simulink model "mission"  (R2019a)
settings: Solver=ode8  StartTime=0.0  StopTime=10000  FixedStep=.1  MaxStep=30  MinStep=1  RelTol=1e-7
PreLoadFcn:
  | load('D:\OneDrive\IonSat X18\SCAO\SIMULINK\Data\SatConstants.mat')
model workspace (MAT data in the model file):
  repartition_matrix = Simulink.Parameter
  repartition_matrix.DataType = 'auto'
  repartition_matrix.Dimensions = [0 0]
  wheel_number = Simulink.Parameter
  wheel_number.Value = 3
  wheel_number.DataType = 'auto'
  wheel_number.Dimensions = [1 1]
undefined symbols (not defined in the file or in its folder): deg, IAU, km, m, mu_Earth, rad, s, sat, X, Y, Z
libraries: sm_lib x19, nesl_utility x16, aerolibutil x15, aerolibconvert2 x12, dspmathops x8, vrlib x5, sharedtransform x5, sharedutil x4, aerolibtransform2 x2, aerolibgravity2 x2, simulink x1, aerolibcelestial x1
(part 1 of 3)
settings Model: SnapshotBufferSize=100  OrderedModelArguments=off  Creator=robin  LastModifiedBy=brice
settings SolverCC: InitialStep=1
settings DataIOCC: SaveFormat=StructureWithTime  SaveOutput=off  SignalLogging=off  DSMLogging=off  SaveTime=off
settings OptimizationCC: DefaultParameterBehavior=Inlined  UseDivisionForNetSlopeComputation=on  GainParamInheritBuiltInType=on  UseFloatMulNetSlope=on  InlineInvariantSignals=on  PassReuseOutputArgsAs=Individual arguments  ZeroExternalMemoryAtStartup=off  ZeroInternalMemoryAtStartup=off  NoFixptDivByZeroProtection=on  EfficientFloat2IntCast=on  LifeSpan=1  OptimizeBlockOrder=speed  DifferentSizesBufferReuse=on
settings DebuggingCC: ParameterTunabilityLossMsg=error
settings HardwareCC: ProdBitPerInt=16  ProdBitPerPointer=8  ProdBitPerSizeT=24  ProdBitPerPtrDiffT=24  ProdLargestAtomicFloat=None  ProdWordSize=8  ProdLongLongMode=on  ProdHWDeviceType=Microchip->PIC18
settings SFSimCC: MATLABDynamicMemAlloc=off
settings RTWCC: SystemTargetFile=ert.tlc  TemplateMakefile=ert_default_tmf  GenerateReport=on  IncludeHyperlinkInReport=on  LaunchReport=on  GenerateTraceInfo=on  GenerateTraceReport=on  GenerateTraceReportSl=on  GenerateTraceReportSf=on  GenerateTraceReportEml=on  GenerateCodeMetricsReport=on
settings CodeAppCC: ForceParamTrailComments=on  IgnoreCustomStorageClasses=off  OperatorAnnotations=on  SimulinkDataObjDesc=on  SFDataObjDesc=on  CustomSymbolStrGlobalVar=rt$N$M  CustomSymbolStrType=$N$M  CustomSymbolStrFcn=$N$M$F  CustomSymbolStrMacro=$N$M  InsertBlockDesc=on
settings ERTTargetCC: TargetLangStandard=C99 (ISO)  GenerateSampleERTMain=on  IncludeMdlTerminateFcn=off  CombineSignalStateStructs=on  SupportAbsoluteTime=off  SupportComplex=off  SupportContinuousTime=on  SupportNonInlinedSFcns=on  InlinedParameterPlacement=NonHierarchical  ERTCustomFileTemplate=example_file_process.tlc  ERTFilePackagingFormat=CompactWithDataFile

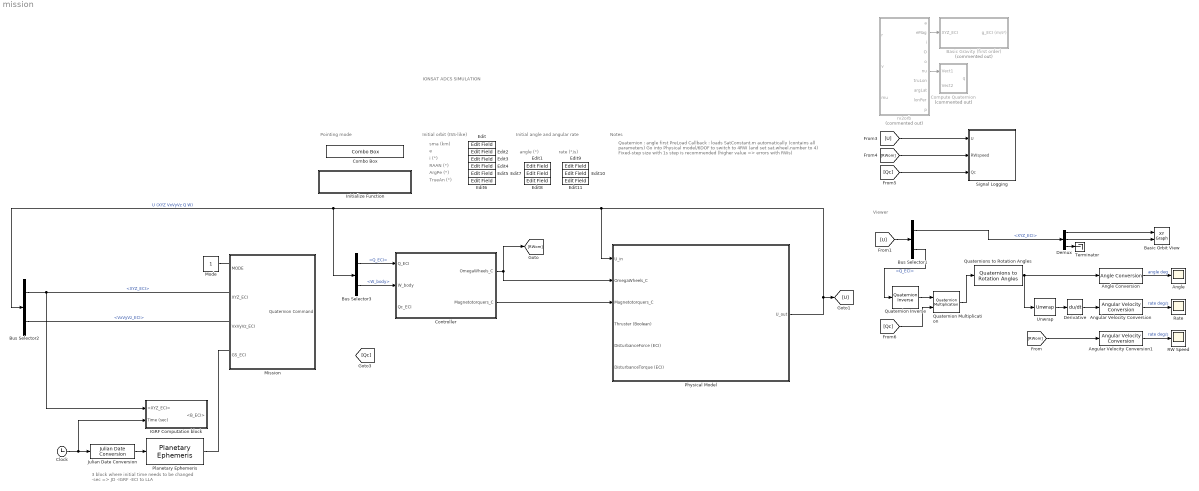
== system mission ==
  note: 3 block where initial time needs to be changed
      | -sec => JD
      | -IGRF
      | -ECI to LLA
  note: IONSAT ADCS SIMULATION
  note: Viewer
  note: Pointing mode
  note: Initial orbit (ISS-like)
  note: sma (km)
  note: e
  note: i (°)
  note: RAAN (°)
  note: ArgPe (°)
  note: TrueAn (°)
  note: Initial angle and angular rate
  note: angle (°)
  note: rate (°/s)
  note: Notes
  note: Quaternion : angle first
      | PreLoad Callback : loads SatConstant.m automatically (contains all parameters)
      | Go into Physical model/6DOF to switch to 4RW (and set sat.wheel.number to 4)
      | Fixed-step size with 1s step is recommended (higher value => errors with RWs)
  Angle : Scope
  Angle Conversion : aerolibconvert2/Angle Conversion  IU=rad  OU=deg
  Angular Velocity Conversion : aerolibconvert2/Angular Velocity Conversion  IU=rad/s  OU=deg/s
      settings: SourceProductName=Aerospace Blockset
  Angular Velocity Conversion1 : aerolibconvert2/Angular Velocity Conversion  IU=rad/s  OU=deg/s
      settings: SourceProductName=Aerospace Blockset
  Basic Gravity (first order) : Subsystem  Commented=on
  Basic Orbit View : simulink/Sinks/XY Graph  xmin=-10000000  xmax=10000000  ymin=-10000000  ymax=10000000  st=-1
  Bus Selector1 : BusSelector  OutputSignals=XYZ_ECI,Q_ECI
  Bus Selector2 : BusSelector  OutputSignals=XYZ_ECI,VxVyVz_ECI
  Bus Selector3 : BusSelector  OutputSignals=Q_ECI,W_body
  Clock : Clock
  Combo Box : ComboBox  LabelPosition=Hide  SelectedLabel=Nadir
      settings: Values={{'Nadir', 'Retrograde', 'Drag', 'Sun', 'Sun Aero'}, [1 5 4 3 2]}
  Compute Quaternion : Subsystem  Commented=on
  Controller : Subsystem  TreatAsAtomicUnit=on  SystemSampleTime=1
  Demux : Demux  Outputs=3
  Derivative : Derivative
  Edit{,1..11} (12 alike) : EditField  LabelPosition=Hide  ShowInitialText=on  Alignment=Center
  IGRF Computation block : Subsystem
  Initialize Function : Subsystem  TreatAsAtomicUnit=on
  Julian Date Conversion : aerolibconvert2/Julian Date Conversion  year=2020  month=January  day=1  hour=0  min=0  sec=0  modflag=off  deltaT=Sec  errorflag=Error
      settings: SourceProductName=Aerospace Blockset  SourceProductBaseCode=AE
  Mission : Subsystem  TreatAsAtomicUnit=on  SystemSampleTime=1
  Mode : Constant  OutDataTypeStr=int8
  Physical Model : Subsystem
  Planetary Ephemeris : aerolibcelestial/Planetary Ephemeris  kmflag=km,km/s  epochflag=Julian date  de=DE405  nCenter=Earth  nTarget=Sun  errorflag=Error  velflag=off
      settings: AttributesFormatString=Ephemeris Data Unavailable  SourceProductName=Aerospace Blockset  SourceProductBaseCode=AE
  Quaternion Inverse : aerolibutil/Quaternion Inverse
      settings: SourceProductName=Aerospace Blockset
  Quaternion Multiplication : aerolibutil/Quaternion Multiplication
  Quaternions to Rotation Angles : sharedtransform/Quaternions to Rotation Angles  rotationOrder=ZYX  aMode=aMode
      settings: SourceProductBaseCode=AE
  RW Speed : Scope
  Rate : Scope
  Signal Logging : Subsystem
  Terminator : Terminator
  Unwrap : dspsigops/Unwrap  tol=pi  running=off
  rv2orb : MATLAB Function  Commented=on  TreatAsAtomicUnit=on
  wires:
  ? -> [Qc], Controller/3(Qc_ECI)  "Quaternion Command"
  Mode/1 -> ?
  Bus Selector2/2 -> ?  "<VxVyVz_ECI>"
  Physical Model/1(U_out) -> Bus Selector3/1, Bus Selector2/1, Physical Model/1(U_in), [U]  "U (XYZ VxVyVz Q W)"
  Controller/2(Magnetotorquers_C) -> Physical Model/3(Magnetotorquers_C)
  Controller/1(OmegaWheels_C) -> [RWom], Physical Model/2(OmegaWheels_C)
  Angle Conversion/1 -> Angle/1  "angle deg"
  Demux/3 -> Terminator/1
  Demux/2 -> Basic Orbit View/2
  Angular Velocity Conversion/1 -> Rate/1  "rate deg/s"
  Bus Selector1/1 -> Demux/1  "<XYZ_ECI>"
  Quaternion Multiplication/1 -> Quaternions to Rotation Angles/1
  Demux/1 -> Basic Orbit View/1
  Derivative/1 -> Angular Velocity Conversion/1
  Quaternions to Rotation Angles/1 -> Unwrap/1, Angle Conversion/1
  Unwrap/1 -> Derivative/1
  Angular Velocity Conversion1/1 -> RW Speed/1  "rate deg/s"
  [RWom] -> Angular Velocity Conversion1/1
  [U] -> Bus Selector1/1
  rv2orb/2(eMag) -> Basic Gravity (first order)/1(XYZ_ECI)
  Bus Selector2/1 -> IGRF Computation block/1(<XYZ_ECI>)  "<XYZ_ECI>"
  rv2orb/6(nu) -> Compute Quaternion/1(Vect1)
  Bus Selector3/1 -> Controller/1(Q_ECI)  "<Q_ECI>"
  Bus Selector3/2 -> Controller/2(W_body)  "<W_body>"
  Julian Date Conversion/1 -> Planetary Ephemeris/1
  Clock/1 -> Julian Date Conversion/1, IGRF Computation block/2(Time (sec))
  Planetary Ephemeris/1 -> ?
  [U] -> Signal Logging/1(U)
  [RWom] -> Signal Logging/2(RWspeed)
  [Qc] -> Signal Logging/3(Qc)
  [Qc] -> Quaternion Multiplication/2
  Quaternion Inverse/1 -> Quaternion Multiplication/1
  Bus Selector1/2 -> Quaternion Inverse/1  "<Q_ECI>"

== system mission/Basic Gravity (first order) ==
  XYZ_ECI : Inport
  Constant : Constant  Value=-mu_Earth
  Constant3 : Constant  Value=3/2
  Divide : Product  Inputs=*/
  Norm : Subsystem
  Product : Product
  Square3 : Math  Operator=pow  SaturateOnIntegerOverflow=on
  g_ECI (m/s²) : Outport  VectorParamsAs1DForOutWhenUnconnected=on
  wires:
  Constant/1 -> Divide/1
  Divide/1 -> Product/2
  Product/1 -> g_ECI (m/s²)/1
  XYZ_ECI/1 -> Norm/1(u), Product/1
  Square3/1 -> Divide/2  "r**3"
  Constant3/1 -> Square3/2
  Norm/1(r**2) -> Square3/1

== system mission/Compute Quaternion ==
  Vect1 : Inport
  Vect2 : Inport  Port=2
  Constant : Constant
  Cross Product : vrlib/Utilities/Cross Product
      settings: SourceProductName=Simulink
  Dot Product : DotProduct  InputSameDT=on  OutDataTypeStr=Inherit: Inherit via internal rule
  Mux : Mux  Inputs=2
  Normalization : dspmathops/Normalization  NormType=2-norm  Bias=1e-10  NormOver=Each column  Dimension=1  roundingMode=Floor  overflowMode=off  accumDataTypeStr=Inherit: Same as product output  accumLastDataTypeStr=Inherit: Same as product output  outputDataTypeStr=Inherit: Same as product output  outputMin=[]  outputMax=[]  outputLastDataTypeStr=Inherit: Same as product output
      settings: SourceProductName=DSP System Toolbox
  Normalization1 : dspmathops/Normalization  NormType=2-norm  Bias=1e-10  NormOver=Each column  Dimension=1  roundingMode=Floor  overflowMode=off  accumDataTypeStr=Inherit: Same as product output  accumLastDataTypeStr=Inherit: Same as product output  outputDataTypeStr=Inherit: Same as product output  outputMin=[]  outputMax=[]  outputLastDataTypeStr=Inherit: Same as product output
      settings: SourceProductName=DSP System Toolbox
  Quaternion Normalize : sharedutil/Quaternion Normalize  aMode=aMode
      settings: SourceProductName=Aerospace Blockset  SourceProductBaseCode=AE
  Sum : Sum  Inputs=|++
  q : Outport  PortDimensions=4
  wires:
  Vect1/1 -> Normalization/1
  Normalization/1 -> Cross Product/1, Dot Product/1
  Vect2/1 -> Normalization1/1
  Normalization1/1 -> Dot Product/2, Cross Product/2
  Cross Product/1 -> Mux/2
  Dot Product/1 -> Sum/1
  Sum/1 -> Mux/1
  Constant/1 -> Sum/2
  Mux/1 -> Quaternion Normalize/1
  Quaternion Normalize/1 -> q/1

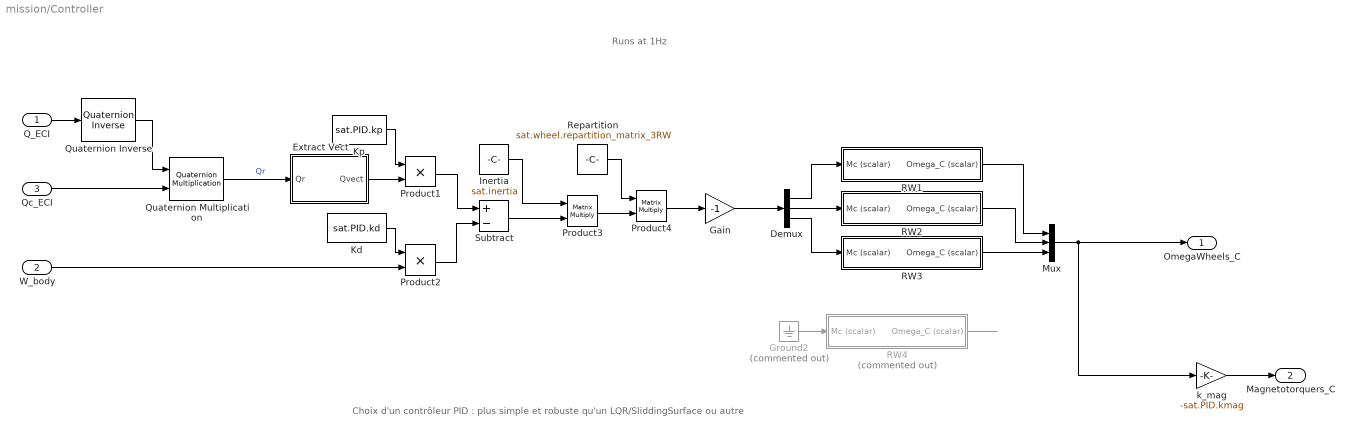
== system mission/Controller ==
  note: Choix d'un contrôleur PID : plus simple et robuste qu'un LQR/SliddingSurface ou autre
  note: Runs at 1Hz
  Q_ECI : Inport
  W_body : Inport  Port=2
  Qc_ECI : Inport  Port=3
  Demux : Demux  Outputs=3
  Extract Vect : Subsystem
  Gain : Gain  Gain=-1
  Ground2 : Ground  Commented=on
  Inertia : Constant  Value=sat.inertia
  Kd : Constant  Value=sat.PID.kd
  Kp : Constant  Value=sat.PID.kp
  Mux : Mux  Inputs=3
  Product1 : Product
  Product2 : Product
  Product3 : Product  Multiplication=Matrix(*)
  Product4 : Product  Multiplication=Matrix(*)
  Quaternion Inverse : aerolibutil/Quaternion Inverse
      settings: SourceProductName=Aerospace Blockset
  Quaternion Multiplication : aerolibutil/Quaternion Multiplication
  RW1 : Subsystem
  RW2 : Subsystem
  RW3 : Subsystem
  RW4 : Subsystem  Commented=on
  Repartition : Constant  Value=sat.wheel.repartition_matrix_3RW
  Subtract : Sum  Inputs=+-
  k_mag : Gain  Gain=-sat.PID.kmag
  OmegaWheels_C : Outport
  Magnetotorquers_C : Outport  Port=2
  wires:
  RW1/1(Omega_C (scalar)) -> Mux/1
  RW2/1(Omega_C (scalar)) -> Mux/2
  RW3/1(Omega_C (scalar)) -> Mux/3
  RW4/1(Omega_C (scalar)) -> ?
  Demux/3 -> RW3/1(Mc (scalar))
  Ground2/1 -> RW4/1(Mc (scalar))
  Qc_ECI/1 -> Quaternion Multiplication/2
  Quaternion Multiplication/1 -> Extract Vect/1(Qr)  "Qr"
  Kp/1 -> Product1/1
  Extract Vect/1(Qvect) -> Product1/2
  W_body/1 -> Product2/2
  Kd/1 -> Product2/1
  Product2/1 -> Subtract/2
  Product1/1 -> Subtract/1
  Subtract/1 -> Product3/2
  Inertia/1 -> Product3/1
  Product3/1 -> Product4/2
  Repartition/1 -> Product4/1
  Demux/2 -> RW2/1(Mc (scalar))
  Demux/1 -> RW1/1(Mc (scalar))
  Product4/1 -> Gain/1
  Q_ECI/1 -> Quaternion Inverse/1
  Quaternion Inverse/1 -> Quaternion Multiplication/1
  Gain/1 -> Demux/1
  k_mag/1 -> Magnetotorquers_C/1
  Mux/1 -> k_mag/1, OmegaWheels_C/1

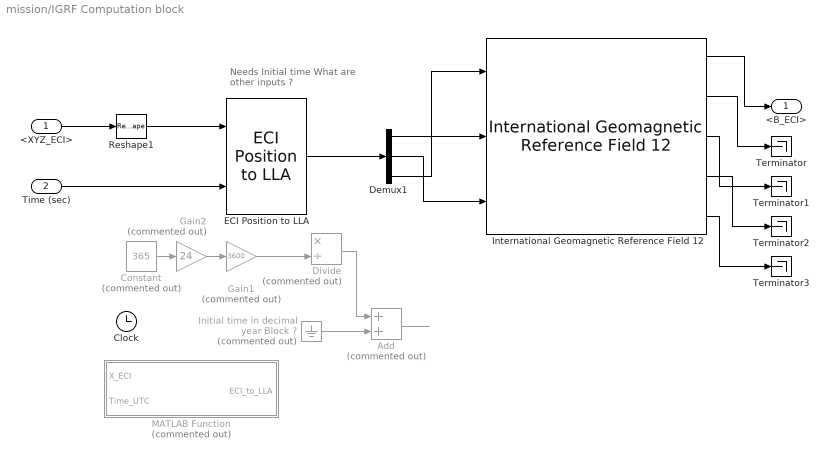
== system mission/IGRF Computation block ==
  note: Needs Initial time
      | What are other inputs ?
  <XYZ_ECI> : Inport
  Time (sec) : Inport  Port=2
  Add : Sum  Commented=on
  Clock : Clock
  Constant : Constant  Commented=on  Value=365
  Demux1 : Demux  Outputs=3
  Divide : Product  Commented=on  Inputs=*/
  ECI Position to LLA : aerolibtransform2/ECI Position to LLA  red=IAU-2000/2006  year=2020  month=January  day=1  hour=0  min=0  sec=0  deltaT=Sec  errorflag=Error  extraparamflag=off  eunits=Metric (MKS)  earthmodel=WGS84  flat=1/298.257223563  eqradius=6378137
      settings: AttributesFormatString=%<red>  SourceProductName=Aerospace Blockset  SourceProductBaseCode=AE
  Gain1 : Gain  Commented=on  Gain=3600
  Gain2 : Gain  Commented=on  Gain=24
  Initial time in decimal year Block ? : Ground  Commented=on
  International Geomagnetic Reference Field 12 : aerolibgravity2/International Geomagnetic Reference Field 12  units=Metric (MKS)  time_in=off  month=January  day=1  year=2020  action=None  sv_out=off
      settings: SourceProductName=Aerospace Blockset  SourceProductBaseCode=AE
  MATLAB Function : MATLAB Function  Commented=on  TreatAsAtomicUnit=on
  Reshape1 : Reshape  OutputDimensionality=Column vector (2-D)
  Terminator{,1..3} (4 alike) : Terminator
  <B_ECI> : Outport
  wires:
  International Geomagnetic Reference Field 12/1 -> <B_ECI>/1
  Demux1/2 -> International Geomagnetic Reference Field 12/3
  Time (sec)/1 -> ECI Position to LLA/2
  ECI Position to LLA/1 -> Demux1/1
  <XYZ_ECI>/1 -> Reshape1/1
  Gain2/1 -> Gain1/1
  Constant/1 -> Gain2/1
  Gain1/1 -> Divide/2
  Add/1 -> ?
  Divide/1 -> Add/1
  Initial time in decimal year Block ?/1 -> Add/2
  Reshape1/1 -> ECI Position to LLA/1
  International Geomagnetic Reference Field 12/3 -> Terminator1/1
  International Geomagnetic Reference Field 12/2 -> Terminator/1
  International Geomagnetic Reference Field 12/4 -> Terminator2/1
  International Geomagnetic Reference Field 12/5 -> Terminator3/1
  Demux1/1 -> International Geomagnetic Reference Field 12/2
  Demux1/3 -> International Geomagnetic Reference Field 12/1

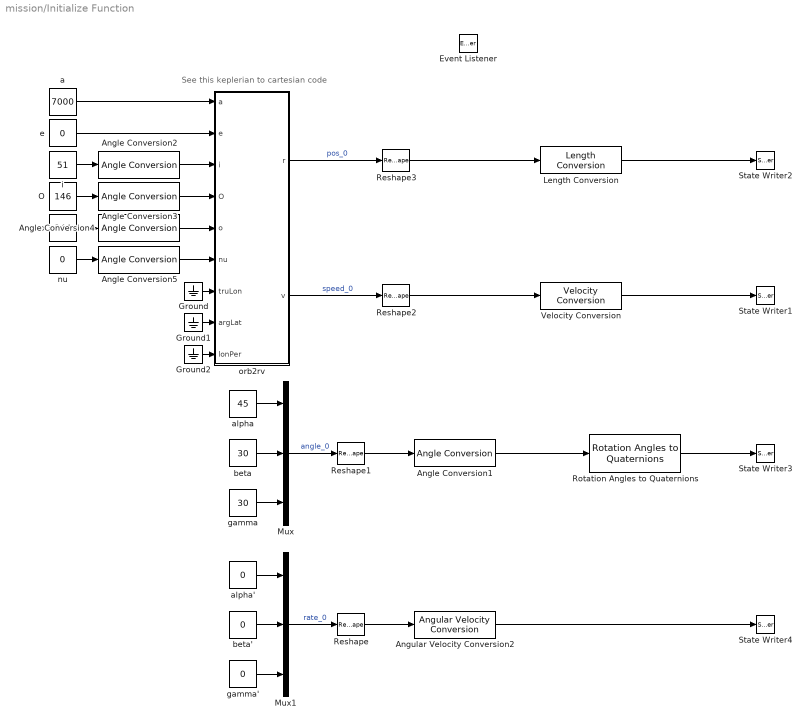
== system mission/Initialize Function ==
  note: See this keplerian to cartesian code
  Angle Conversion{1..5} (5 alike) : aerolibconvert2/Angle Conversion  IU=deg  OU=rad
  Angular Velocity Conversion2 : aerolibconvert2/Angular Velocity Conversion  IU=deg/s  OU=rad/s
      settings: SourceProductName=Aerospace Blockset
  Event Listener : EventListener  DisableCoverage=on  EventName=reset
  Ground : Ground
  Ground1 : Ground
  Ground2 : Ground
  Length Conversion : aerolibconvert2/Length Conversion  IU=km  OU=m
  Mux : Mux  Inputs=3
  Mux1 : Mux  Inputs=3
  O : Constant  Value=146
  Reshape{,1..3} (4 alike) : Reshape  OutputDimensionality=Column vector (2-D)
  Rotation Angles to Quaternions : sharedtransform/Rotation Angles to Quaternions  rotationOrder=ZYX  aMode=aMode
      settings: SourceProductName=Aerospace Blockset  SourceProductBaseCode=AE
  State Writer1 : StateWriter  StateOwnerBlock=../../Physical Model/6DOF in ECI frame/Integrator_speed
  State Writer2 : StateWriter  StateOwnerBlock=../../Physical Model/6DOF in ECI frame/Integrator_pos
  State Writer3 : StateWriter  StateOwnerBlock=../../Physical Model/6DOF in ECI frame/Compute Q_ECI/Integrator_quat
  State Writer4 : StateWriter  StateOwnerBlock=../../Physical Model/6DOF in ECI frame/Integrator_rate
  Velocity Conversion : aerolibconvert2/Velocity Conversion  IU=km/s  OU=m/s
  a : Constant  Value=7000
  alpha : Constant  Value=45
  alpha' : Constant  Value=0
  beta : Constant  Value=30
  beta' : Constant  Value=0
  e : Constant  Value=0
  gamma : Constant  Value=30
  gamma' : Constant  Value=0
  i : Constant  Value=51
  nu : Constant  Value=0
  o : Constant  Value=344
  orb2rv : MATLAB Function  TreatAsAtomicUnit=on
  wires:
  Angular Velocity Conversion2/1 -> State Writer4/1
  Angle Conversion1/1 -> Rotation Angles to Quaternions/1
  orb2rv/1(r) -> Reshape3/1  "pos_0"
  Mux1/1 -> Reshape/1  "rate_0"
  Mux/1 -> Reshape1/1  "angle_0"
  orb2rv/2(v) -> Reshape2/1  "speed_0"
  Rotation Angles to Quaternions/1 -> State Writer3/1
  Reshape/1 -> Angular Velocity Conversion2/1
  Reshape1/1 -> Angle Conversion1/1
  Reshape2/1 -> Velocity Conversion/1
  Reshape3/1 -> Length Conversion/1
  a/1 -> orb2rv/1(a)
  e/1 -> orb2rv/2(e)
  i/1 -> Angle Conversion2/1
  O/1 -> Angle Conversion3/1
  o/1 -> Angle Conversion4/1
  nu/1 -> Angle Conversion5/1
  Angle Conversion2/1 -> orb2rv/3(i)
  Angle Conversion3/1 -> orb2rv/4(O)
  Angle Conversion4/1 -> orb2rv/5(o)
  Angle Conversion5/1 -> orb2rv/6(nu)
  Ground/1 -> orb2rv/7(truLon)
  Ground1/1 -> orb2rv/8(argLat)
  Ground2/1 -> orb2rv/9(lonPer)
  Length Conversion/1 -> State Writer2/1
  Velocity Conversion/1 -> State Writer1/1
  alpha/1 -> Mux/1
  beta/1 -> Mux/2
  gamma/1 -> Mux/3
  alpha'/1 -> Mux1/1
  gamma'/1 -> Mux1/3
  beta'/1 -> Mux1/2

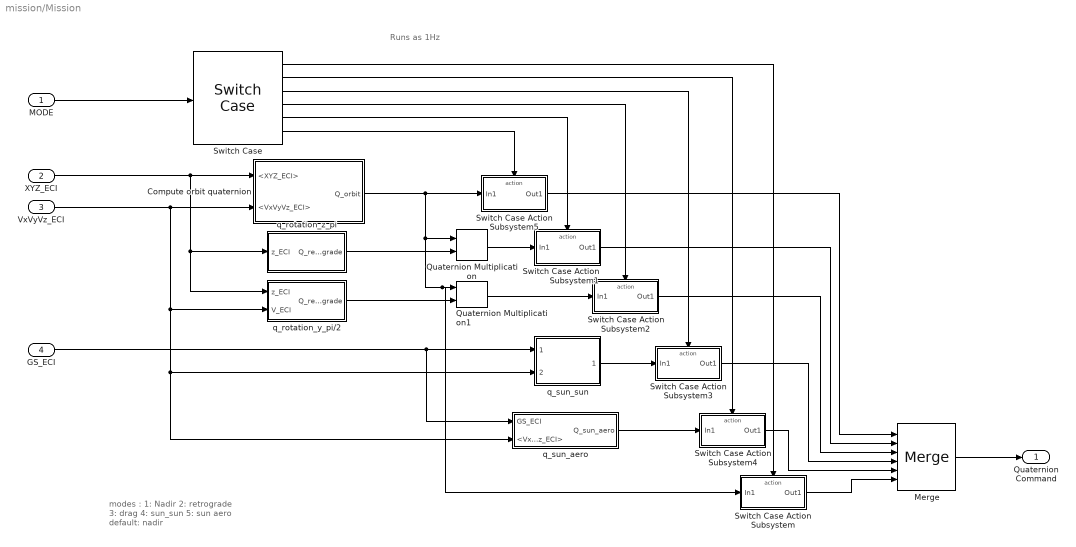
== system mission/Mission ==
  note: modes :
      | 1: Nadir
      | 2: retrograde
      | 3: drag
      | 4: sun_sun
      | 5: sun aero
      | default: nadir
  note: Runs as 1Hz
  MODE : Inport  OutMin=1  OutMax=100  OutDataTypeStr=int8
  XYZ_ECI : Inport  Port=2
  VxVyVz_ECI : Inport  Port=3
  GS_ECI : Inport  Port=4
  Compute orbit quaternion : Subsystem
  Merge : Merge  Inputs=6
  Quaternion Multiplication : aerolibutil/Quaternion Multiplication
  Quaternion Multiplication1 : aerolibutil/Quaternion Multiplication
  Switch Case : SwitchCase  CaseConditions={1, 2, 3, 4, 5}
  Switch Case Action Subsystem : Subsystem  TreatAsAtomicUnit=on
  Switch Case Action Subsystem1 : Subsystem  TreatAsAtomicUnit=on
  Switch Case Action Subsystem2 : Subsystem  TreatAsAtomicUnit=on
  Switch Case Action Subsystem3 : Subsystem  TreatAsAtomicUnit=on
  Switch Case Action Subsystem4 : Subsystem  TreatAsAtomicUnit=on
  Switch Case Action Subsystem5 : Subsystem  TreatAsAtomicUnit=on
  q_rotation_y_pi/2 : Subsystem
  q_rotation_z_pi : Subsystem
  q_sun_aero : Subsystem
  q_sun_sun : Subsystem
  Quaternion Command : Outport
  wires:
  q_rotation_y_pi/2/1(Q_retrograde) -> Quaternion Multiplication1/2
  Switch Case/6 -> Switch Case Action Subsystem5/Action
  Switch Case/3 -> Switch Case Action Subsystem3/Action
  Switch Case/1 -> Switch Case Action Subsystem/Action
  MODE/1 -> Switch Case/1
  Switch Case Action Subsystem2/1(Out1) -> Merge/3
  Switch Case Action Subsystem4/1(Out1) -> Merge/5
  Quaternion Multiplication1/1 -> Switch Case Action Subsystem2/1(In1)
  GS_ECI/1 -> q_sun_aero/1(GS_ECI), q_sun_sun/1(<VxVyVz_ECI>)
  Switch Case Action Subsystem3/1(Out1) -> Merge/4
  XYZ_ECI/1 -> q_rotation_y_pi/2/1(z_ECI), q_rotation_z_pi/1(z_ECI), Compute orbit quaternion/1(<XYZ_ECI>)
  Switch Case/4 -> Switch Case Action Subsystem2/Action
  Compute orbit quaternion/1(Q_orbit) -> Switch Case Action Subsystem/1(In1), Quaternion Multiplication1/1, Quaternion Multiplication/1, Switch Case Action Subsystem5/1(In1)
  Switch Case Action Subsystem/1(Out1) -> Merge/6
  Quaternion Multiplication/1 -> Switch Case Action Subsystem1/1(In1)
  q_rotation_z_pi/1(Q_retrograde) -> Quaternion Multiplication/2
  Switch Case/5 -> Switch Case Action Subsystem1/Action
  Switch Case Action Subsystem1/1(Out1) -> Merge/2
  q_sun_aero/1(Q_sun_aero) -> Switch Case Action Subsystem4/1(In1)
  Merge/1 -> Quaternion Command/1
  Switch Case/2 -> Switch Case Action Subsystem4/Action
  Switch Case Action Subsystem5/1(Out1) -> Merge/1
  q_sun_sun/1(Q_sun_sun) -> Switch Case Action Subsystem3/1(In1)
  VxVyVz_ECI/1 -> q_sun_aero/2(<VxVyVz_ECI>), q_sun_sun/2(GS_ECI), q_rotation_y_pi/2/2(V_ECI), Compute orbit quaternion/2(<VxVyVz_ECI>)

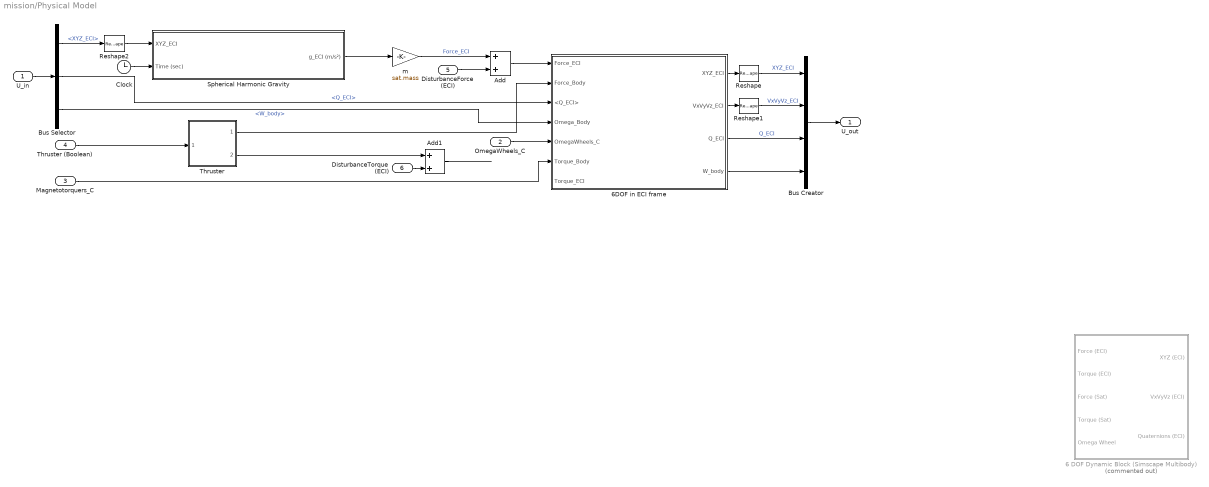
== system mission/Physical Model ==
  U_in : Inport
  OmegaWheels_C : Inport  Port=2
  Magnetotorquers_C : Inport  Port=3
  Thruster (Boolean) : Inport  Port=4
  DisturbanceForce (ECI) : Inport  Port=5
  DisturbanceTorque (ECI) : Inport  Port=6
  6 DOF Dynamic Block (Simscape Multibody) : Subsystem  Commented=on
  6DOF in ECI frame : Subsystem
  Add : Sum
  Add1 : Sum
  Bus Creator : BusCreator  Inputs=4
  Bus Selector : BusSelector  OutputSignals=XYZ_ECI,Q_ECI,W_body
  Clock : Clock
  Reshape : Reshape
  Reshape1 : Reshape
  Reshape2 : Reshape  OutputDimensionality=Column vector (2-D)
  Spherical Harmonic Gravity : Subsystem  TreatAsAtomicUnit=on  SystemSampleTime=1
  Thruster : Subsystem
  m : Gain  Gain=sat.mass
  U_out : Outport
  wires:
  Bus Selector/1 -> Reshape2/1  "<XYZ_ECI>"
  Spherical Harmonic Gravity/1(g_ECI (m/s²)) -> m/1
  Thruster (Boolean)/1 -> Thruster/1(On/Off (Boolean))
  U_in/1 -> Bus Selector/1
  Bus Creator/1 -> U_out/1
  Bus Selector/2 -> 6DOF in ECI frame/3(<Q_ECI>)  "<Q_ECI>"
  OmegaWheels_C/1 -> 6DOF in ECI frame/5(OmegaWheels_C)
  6DOF in ECI frame/3(Q_ECI) -> Bus Creator/3  "Q_ECI"
  6DOF in ECI frame/1(XYZ_ECI) -> Reshape/1
  6DOF in ECI frame/2(VxVyVz_ECI) -> Reshape1/1
  m/1 -> Add/1  "Force_ECI"
  Add/1 -> 6DOF in ECI frame/1(Force_ECI)
  Thruster/1(Force (G_sat)) -> 6DOF in ECI frame/2(Force_Body)
  Magnetotorquers_C/1 -> 6DOF in ECI frame/6(Torque_Body)
  Thruster/2(Moment (G_sat)) -> Add1/1
  Add1/1 -> ?
  DisturbanceForce (ECI)/1 -> Add/2
  DisturbanceTorque (ECI)/1 -> Add1/2
  Reshape/1 -> Bus Creator/1  "XYZ_ECI"
  Reshape1/1 -> Bus Creator/2  "VxVyVz_ECI"
  Reshape2/1 -> Spherical Harmonic Gravity/1(XYZ_ECI)
  6DOF in ECI frame/4(W_body) -> Bus Creator/4
  Bus Selector/3 -> 6DOF in ECI frame/4("Omega_Body ")  "<W_body>"
  Clock/1 -> Spherical Harmonic Gravity/2(Time (sec))

== system mission/Signal Logging ==
  U : Inport
  RWspeed : Inport  Port=2
  Qc : Inport  Port=3
  Bus Selector4 : BusSelector  OutputSignals=XYZ_ECI,VxVyVz_ECI,Q_ECI,W_body
  To Workspace : ToWorkspace  VariableName=sat_pos  SaveFormat=Timeseries  SampleTime=-1
      settings: Save2DSignal=2-D array (concatenate along first dimension)
  To Workspace1 : ToWorkspace  VariableName=sat_speed  SaveFormat=Timeseries  SampleTime=-1
      settings: Save2DSignal=2-D array (concatenate along first dimension)
  To Workspace2 : ToWorkspace  VariableName=sat_Q  SaveFormat=Timeseries  SampleTime=-1
      settings: Save2DSignal=2-D array (concatenate along first dimension)
  To Workspace3 : ToWorkspace  VariableName=sat_omega  SaveFormat=Timeseries  SampleTime=-1
      settings: Save2DSignal=2-D array (concatenate along first dimension)
  To Workspace4 : ToWorkspace  VariableName=RW_omega  SaveFormat=Timeseries  SampleTime=-1
      settings: Save2DSignal=2-D array (concatenate along first dimension)
  To Workspace5 : ToWorkspace  VariableName=sat_Qc  SaveFormat=Timeseries  SampleTime=-1
      settings: Save2DSignal=2-D array (concatenate along first dimension)
  wires:
  Bus Selector4/3 -> To Workspace2/1  "<Q_ECI>"
  Bus Selector4/4 -> To Workspace3/1  "<W_body>"
  U/1 -> Bus Selector4/1
  Bus Selector4/2 -> To Workspace1/1  "<VxVyVz_ECI>"
  RWspeed/1 -> To Workspace4/1
  Bus Selector4/1 -> To Workspace/1  "<XYZ_ECI>"
  Qc/1 -> To Workspace5/1

== system mission/Basic Gravity (first order)/Norm ==
  u : Inport
  Abs : Abs
  Add : Sum  Inputs=+++
  Demux1 : Demux  Outputs=3
  Square : Math  Operator=square  SaturateOnIntegerOverflow=on
  Square1 : Math  Operator=square  SaturateOnIntegerOverflow=on
  Square2 : Math  Operator=square  SaturateOnIntegerOverflow=on
  r**2 : Outport
  wires:
  Demux1/2 -> Square1/1
  Add/1 -> r**2/1  "r**2"
  Square/1 -> Add/1
  u/1 -> Abs/1
  Demux1/1 -> Square/1
  Demux1/3 -> Square2/1
  Abs/1 -> Demux1/1
  Square2/1 -> Add/3
  Square1/1 -> Add/2

== system mission/Controller/Extract Vect ==
  Qr : Inport
  Demux : Demux
  Mux1 : Mux  Inputs=3
  Product : Product
  Sign : Signum
  Qvect : Outport
  wires:
  Demux/2 -> Mux1/1
  Demux/4 -> Mux1/3
  Demux/3 -> Mux1/2
  Demux/1 -> Sign/1
  Qr/1 -> Demux/1
  Mux1/1 -> Product/2
  Product/1 -> Qvect/1
  Sign/1 -> Product/1

== system mission/Controller/RW1 ==
  note: Entrées:
      | - Moment de commande (déjà projeté sur l'axe de la roue...)
      | Sorties:
      | - Omega de commande à appliquer
  Mc (scalar) : Inport
  Divide : Product  Inputs=*/
  Integrator : Integrator
  Saturation_speed : Saturate  UpperLimit=sat.wheel.max_speed  LowerLimit=- sat.wheel.max_speed
  Torque_sat : Saturate  UpperLimit=sat.wheel.max_torque  LowerLimit=- sat.wheel.max_torque
  Wheel Inertia : Constant  Value=sat.wheel.max_sigma/sat.wheel.max_speed
  Omega_C (scalar) : Outport  VectorParamsAs1DForOutWhenUnconnected=on
  wires:
  Wheel Inertia/1 -> Divide/2
  Divide/1 -> Integrator/1  "dw/dt"
  Integrator/1 -> Saturation_speed/1
  Torque_sat/1 -> Divide/1  "Torque (scal)"
  Saturation_speed/1 -> Omega_C (scalar)/1
  Mc (scalar)/1 -> Torque_sat/1

== system mission/Controller/RW2 ==
  note: Entrées:
      | - Moment de commande (déjà projeté sur l'axe de la roue...)
      | Sorties:
      | - Omega de commande à appliquer
  Mc (scalar) : Inport
  Divide : Product  Inputs=*/
  Integrator : Integrator
  Saturation_speed : Saturate  UpperLimit=sat.wheel.max_speed  LowerLimit=- sat.wheel.max_speed
  Torque_sat : Saturate  UpperLimit=sat.wheel.max_torque  LowerLimit=- sat.wheel.max_torque
  Wheel Inertia : Constant  Value=sat.wheel.max_sigma/sat.wheel.max_speed
  Omega_C (scalar) : Outport  VectorParamsAs1DForOutWhenUnconnected=on
  wires:
  Wheel Inertia/1 -> Divide/2
  Divide/1 -> Integrator/1  "dw/dt"
  Integrator/1 -> Saturation_speed/1
  Torque_sat/1 -> Divide/1  "Torque (scal)"
  Saturation_speed/1 -> Omega_C (scalar)/1
  Mc (scalar)/1 -> Torque_sat/1

== system mission/Controller/RW3 ==
  note: Entrées:
      | - Moment de commande (déjà projeté sur l'axe de la roue...)
      | Sorties:
      | - Omega de commande à appliquer
  Mc (scalar) : Inport
  Divide : Product  Inputs=*/
  Integrator : Integrator
  Saturation_speed : Saturate  UpperLimit=sat.wheel.max_speed  LowerLimit=- sat.wheel.max_speed
  Torque_sat : Saturate  UpperLimit=sat.wheel.max_torque  LowerLimit=- sat.wheel.max_torque
  Wheel Inertia : Constant  Value=sat.wheel.max_sigma/sat.wheel.max_speed
  Omega_C (scalar) : Outport  VectorParamsAs1DForOutWhenUnconnected=on
  wires:
  Wheel Inertia/1 -> Divide/2
  Divide/1 -> Integrator/1  "dw/dt"
  Integrator/1 -> Saturation_speed/1
  Torque_sat/1 -> Divide/1  "Torque (scal)"
  Saturation_speed/1 -> Omega_C (scalar)/1
  Mc (scalar)/1 -> Torque_sat/1

== system mission/Controller/RW4 ==
  note: Entrées:
      | - Moment de commande (déjà projeté sur l'axe de la roue...)
      | Sorties:
      | - Omega de commande à appliquer
  Mc (scalar) : Inport
  Divide : Product  Inputs=*/
  Integrator : Integrator
  Saturation_speed : Saturate  UpperLimit=sat.wheel.max_speed  LowerLimit=- sat.wheel.max_speed
  Torque_sat : Saturate  UpperLimit=sat.wheel.max_torque  LowerLimit=- sat.wheel.max_torque
  Wheel Inertia : Constant  Value=sat.wheel.max_sigma/sat.wheel.max_speed
  Omega_C (scalar) : Outport  VectorParamsAs1DForOutWhenUnconnected=on
  wires:
  Mc (scalar)/1 -> Torque_sat/1
  Wheel Inertia/1 -> Divide/2
  Divide/1 -> Integrator/1  "dw/dt"
  Integrator/1 -> Saturation_speed/1
  Torque_sat/1 -> Divide/1  "Torque (scal)"
  Saturation_speed/1 -> Omega_C (scalar)/1

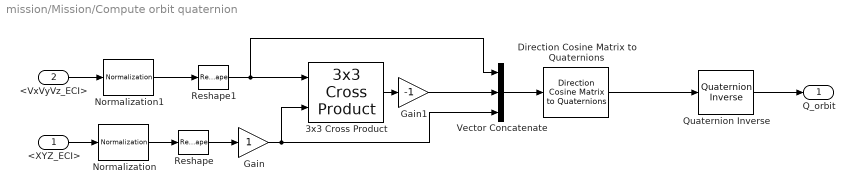
== system mission/Mission/Compute orbit quaternion ==
  <XYZ_ECI> : Inport
  <VxVyVz_ECI> : Inport  Port=2
  3x3 Cross Product : sharedutil/3x3 Cross Product  aMode=aMode
      settings: SourceProductBaseCode=AE
  Direction Cosine Matrix to Quaternions : sharedtransform/Direction Cosine Matrix  to Quaternions  aMode=0  action=None  tolerance=eps(2)
      settings: SourceProductName=Aerospace Blockset  SourceProductBaseCode=AE
  Gain : Gain
  Gain1 : Gain  Gain=-1
  Normalization : dspmathops/Normalization  NormType=2-norm  Bias=1e-10  NormOver=Each column  Dimension=1  roundingMode=Floor  overflowMode=off  accumDataTypeStr=Inherit: Same as product output  accumLastDataTypeStr=Inherit: Same as product output  outputDataTypeStr=Inherit: Same as product output  outputMin=[]  outputMax=[]  outputLastDataTypeStr=Inherit: Same as product output
      settings: SourceProductName=DSP System Toolbox
  Normalization1 : dspmathops/Normalization  NormType=2-norm  Bias=1e-10  NormOver=Each column  Dimension=1  roundingMode=Floor  overflowMode=off  accumDataTypeStr=Inherit: Same as product output  accumLastDataTypeStr=Inherit: Same as product output  outputDataTypeStr=Inherit: Same as product output  outputMin=[]  outputMax=[]  outputLastDataTypeStr=Inherit: Same as product output
      settings: SourceProductName=DSP System Toolbox
  Quaternion Inverse : aerolibutil/Quaternion Inverse
      settings: SourceProductName=Aerospace Blockset
  Reshape : Reshape  OutputDimensionality=Column vector (2-D)
  Reshape1 : Reshape  OutputDimensionality=Column vector (2-D)
  Vector Concatenate : Concatenate  NumInputs=3  Mode=Multidimensional array  ConcatenateDimension=2
  Q_orbit : Outport
  wires:
  Normalization/1 -> Reshape/1
  Normalization1/1 -> Reshape1/1
  <VxVyVz_ECI>/1 -> Normalization1/1
  Reshape1/1 -> 3x3 Cross Product/1, Vector Concatenate/1
  <XYZ_ECI>/1 -> Normalization/1
  Reshape/1 -> Gain/1
  Gain/1 -> 3x3 Cross Product/2, Vector Concatenate/3
  Direction Cosine Matrix to Quaternions/1 -> Quaternion Inverse/1
  3x3 Cross Product/1 -> Gain1/1
  Gain1/1 -> Vector Concatenate/2
  Quaternion Inverse/1 -> Q_orbit/1
  Vector Concatenate/1 -> Direction Cosine Matrix to Quaternions/1

== system mission/Mission/Switch Case Action Subsystem ==
  In1 : Inport
  Action Port : ActionPort  ActionPortLabel=case [ 1 ]:
  Out1 : Outport
  wires:
  In1/1 -> Out1/1

== system mission/Mission/Switch Case Action Subsystem1 ==
  In1 : Inport
  Action Port : ActionPort  ActionPortLabel=case [ 5 ]:
  Out1 : Outport
  wires:
  In1/1 -> Out1/1

== system mission/Mission/Switch Case Action Subsystem2 ==
  In1 : Inport
  Action Port : ActionPort  ActionPortLabel=case [ 4 ]:
  Out1 : Outport
  wires:
  In1/1 -> Out1/1

== system mission/Mission/Switch Case Action Subsystem3 ==
  In1 : Inport
  Action Port : ActionPort  ActionPortLabel=case [ 3 ]:
  Out1 : Outport
  wires:
  In1/1 -> Out1/1

== system mission/Mission/Switch Case Action Subsystem4 ==
  In1 : Inport
  Action Port : ActionPort  ActionPortLabel=case [ 2 ]:
  Out1 : Outport
  wires:
  In1/1 -> Out1/1

== system mission/Mission/Switch Case Action Subsystem5 ==
  In1 : Inport
  Action Port : ActionPort  ActionPortLabel=default:
  Out1 : Outport
  wires:
  In1/1 -> Out1/1

== system mission/Mission/q_rotation_y_pi//2 ==
  z_ECI : Inport
  V_ECI : Inport  Port=2
  Cross Product : vrlib/Utilities/Cross Product
      settings: SourceProductName=Simulink
  Product : Product
  Reshape1 : Reshape  OutputDimensionality=Column vector (2-D)
  Vector Concatenate1 : Concatenate  Mode=Multidimensional array
  cos pi/4 : Constant  Value=[sqrt(2)]
  sin pi/4 : Constant  Value=sqrt(2)
  Q_retrograde : Outport
  wires:
  cos pi/4/1 -> Vector Concatenate1/1
  Vector Concatenate1/1 -> Q_retrograde/1
  sin pi/4/1 -> Product/2
  z_ECI/1 -> Cross Product/1
  V_ECI/1 -> Cross Product/2
  Cross Product/1 -> Product/1  "y"
  Reshape1/1 -> Vector Concatenate1/2
  Product/1 -> Reshape1/1

== system mission/Mission/q_rotation_z_pi ==
  z_ECI : Inport
  Product : Product
  Reshape1 : Reshape  OutputDimensionality=Column vector (2-D)
  Vector Concatenate1 : Concatenate  Mode=Multidimensional array
  cos pi/2 : Constant  Value=[0]
  sin pi/2 : Constant
  Q_retrograde : Outport
  wires:
  cos pi/2/1 -> Vector Concatenate1/1
  Vector Concatenate1/1 -> Q_retrograde/1
  sin pi/2/1 -> Product/2
  z_ECI/1 -> Product/1
  Product/1 -> Reshape1/1
  Reshape1/1 -> Vector Concatenate1/2

== system mission/Mission/q_sun_aero ==
  GS_ECI : Inport
  <VxVyVz_ECI> : Inport  Port=2
  Subsystem : Subsystem
  Q_sun_aero : Outport
  wires:
  <VxVyVz_ECI>/1 -> Subsystem/1(<VxVyVz_ECI>)
  Subsystem/1(Q_sun_aero) -> Q_sun_aero/1
  GS_ECI/1 -> Subsystem/2(GS_ECI)

== system mission/Mission/q_sun_sun ==
  <VxVyVz_ECI> : Inport
  GS_ECI : Inport  Port=2
  Subsystem1 : Subsystem
  Q_sun_sun : Outport
  wires:
  GS_ECI/1 -> Subsystem1/1(GS_ECI)
  <VxVyVz_ECI>/1 -> Subsystem1/2(VxVyVz_ECI)
  Subsystem1/1(Q_sun_aero1) -> Q_sun_sun/1
